simulink model "BaseFile"  (R2012b)
settings: Solver=ode45  StartTime=0.0  StopTime=10.0  RelTol=1e-3
libraries: simulink x1
settings Model: Creator=Kushal  LastModifiedBy=Kushal

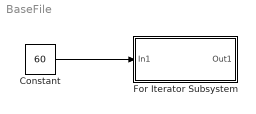
== system BaseFile ==
  Constant : Constant  Value=60
  For Iterator Subsystem : Subsystem  TreatAsAtomicUnit=on
  wires:
  Constant/1 -> For Iterator Subsystem/1(In1)

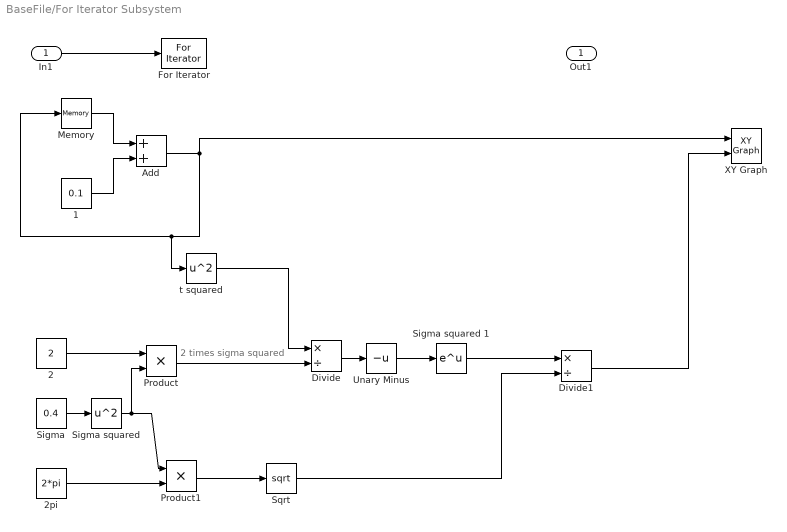
== system BaseFile/For Iterator Subsystem ==
  note: 2 times sigma squared
  In1 : Inport
  1 : Constant  Value=0.1
  2 : Constant  Value=2
  "2pi " : Constant  Value=2*pi
  Add : Sum
  Divide : Product  Inputs=*/
  Divide1 : Product  Inputs=*/
  For Iterator : ForIterator  ResetStates=reset  IterationSource=external
  Memory : Memory  X0=-3.1  InheritSampleTime=on
  Product : Product  RndMeth=Zero
  Product1 : Product  RndMeth=Zero
  "Sigma " : Constant  Value=0.4
  "Sigma squared " : Math  Operator=square  SaturateOnIntegerOverflow=on
  Sigma squared 1 : Math  SaturateOnIntegerOverflow=on
  Sqrt : Sqrt  SaturateOnIntegerOverflow=on
  Unary Minus : UnaryMinus
  XY Graph : simulink/Sinks/XY Graph  xmin=-3  xmax=3  ymin=0  ymax=1  st=-1
  "t squared " : Math  Operator=square  SaturateOnIntegerOverflow=on
  Out1 : Outport
  wires:
  "Sigma "/1 -> "Sigma squared "/1
  "t squared "/1 -> Divide/1
  Product/1 -> Divide/2
  Sigma squared 1/1 -> Divide1/1
  2/1 -> Product/1
  "Sigma squared "/1 -> Product1/1, Product/2
  "2pi "/1 -> Product1/2
  Product1/1 -> Sqrt/1
  Sqrt/1 -> Divide1/2
  Unary Minus/1 -> Sigma squared 1/1
  Divide/1 -> Unary Minus/1
  In1/1 -> For Iterator/1
  Memory/1 -> Add/1
  1/1 -> Add/2
  Divide1/1 -> XY Graph/2
  Add/1 -> "t squared "/1, Memory/1, XY Graph/1
